simulink model "IEEE9-WT-PV"  (R2024a)
settings: Solver=FixedStepDiscrete  StartTime=0.0  StopTime=Tend  RelTol=1e-3
values from neighbouring files (symbols this model uses):
  beta_0 = 0    [data_WT.m]
  C_4 = 0.1670*C_b    (= 1.00487241952e-06)    [main.m]
  C_6 = 0.2835*C_b    (= 1.70587623314e-06)    [main.m]
  C_8 = 0.2275*C_b    (= 1.36891302659e-06)    [main.m]
  C_dc = 2*S_LV_base*H_DC_base/V_dc_base^2    (= 0.478267523722)    [data_WT.m]    (also in main.m = 1.6)
  C_f = C_f_pu*C_LV_base    (= 0.001461477898)    [data_WT.m]    (also in main.m = 0.00530516476973)
  f_b = 50    [data_WT.m]    (also in main.m)
  fdr_m = 0.05    [main.m]
  fdr_q = 0.01    [main.m]
  G_diff = ss(c2d(s/(20e-3/3*s+1),T_s_cont,'tustin'))    [data_WT.m]
  G_lowpass_disc = ss(c2d(G_lowpass,T_s_cont,'tustin'))    [data_WT.m]
  G_lowpass_disc_1khz = ss(c2d(G_lowpass_1khz,T_s_cont,'tustin'))    [data_WT.m]
  G_setpoint_lowpass_disc = ss(c2d(ss(1/(0.1*s+1)),T_s_cont,'tustin'))    [main.m]
  G_sm_dis = ss(c2d(G_cont_sm,T_s_sim,'tustin'))    [main.m]
  GSC_theta0 = -45.0572/180*pi*0-60/180*pi    (= -1.0471975512)    [data_WT.m]
  I0_total1 = Npar1*I0    (= 7.7895e-08)    [data_PV.m]
  I_GSC_base = S_GSC_base/V_LV_base    (= 30303.030303)    [data_WT.m]
  I_PMSG_0 = T_park(0)^-1*[Z_PMSG^-1*V_LV_base*sqrt(2/3)*([cos(RSC_theta0);sin(RSC_theta0)]-[cos(PMSG_theta0);sin(PMSG_theta0)]);0]    [data_WT.m]
  IL_total1 = Npar1*IL    (= 50459)    [data_PV.m]
  Ipv_scmax1 = Npar1*Ipv_sc    (= 50300)    [data_PV.m]
  island_q = [-0.1312   -0.0230   -0.0343]    [main.m]
  island_Vdc = [1 1.2853    Vpv_mppmax2/Vdc_n]    [main.m]
  island_Vdc_r = [1 1.3430 1.4716]    [main.m]
  island_Vm = [1 1 1]    [main.m]
  J_PMSG_WT_MS = 2*H_PMSGWT_LS*S_PMSG_base/(2*pi*f_b)^2    (= 630.526507942)    [data_WT.m]
  k_p_GSC = 0.02    [data_WT.m]
  k_p_MSC = k_p_GSC    (= 0.02)    [data_WT.m]
  k_theta_GSC = 0.1    [data_WT.m]
  k_theta_MSC = 2/0.6    (= 3.33333333333)    [data_WT.m]
  K_WT_ff_i = 1    [main.m]
  K_WT_ff_v = 1    [main.m]
  K_WT_i_i = 0.79    [main.m]
  K_WT_i_v = 0.69    [main.m]
  K_WT_p_i = 2.1    [main.m]
  K_WT_p_v = 0.15    [main.m]
  Kff_v = 1    [main.m]
  Kffpv_i = 1    [main.m]
  Kp_beta = 270*0    (= 0)    [data_WT.m]
  Kpvi_i1 = Ki_i*Vpv_m/Ipv_b_LV    [main.m]
  Kpvi_v1 = Ki_v*Ipv_b_LV/Vpv_m    [main.m]
  Kpvp_i1 = Kp_i*Vpv_m/Ipv_b_LV    [main.m]
  Kpvp_v1 = Kp_v*Ipv_b_LV/Vpv_m    [main.m]
  L1_pu = 1*0.0186/m    (= 0.000186)    [main.m]
  L_45 = L_lines(2)    [main.m]
  L_56 = L_lines(3)    [main.m]
  L_67 = L_lines(5)    [main.m]
  L_78 = L_lines(6)    [main.m]
  L_89 = L_lines(8)    [main.m]
  L_94 = L_lines(9)    [main.m]
  L_f = L_f_pu*L_LV_base    (= 3.46639466054e-05)    [data_WT.m]    (also in main.m = 9.54929658551e-06)
  L_PMSG = L_PMSG_PU*L_LV_base    (= 3.46639466054e-05)    [data_WT.m]
  main_p = 0.575    [main.m]
  mpv_dc1 = fdr*kg1*w_b/Vdc_n    [main.m]
  mpv_dc1_r = fdr*kg1_r*w_b/Vdc_n    [main.m]
  mpv_p1 = fdr_p/Vdc_n*w_b    [main.m]
  mpv_q1 = fdr_q*Vpv_m/S_b    [main.m]
  Notch_w_10khz = ss(c2d((s^2+w0_f10khz^2)/(s^2+w0_f10khz/Q_f10khz*s+w0_f10khz^2),T_s_sim,'tustin'))    [data_WT.m]
  omega_base = 2*pi*f_b    (= 314.159265359)    [data_WT.m]    (also in main.m)
  omega_wt = 1.4    [data_WT.m]
  R1_pu = 1*0.00734/m    (= 7.34e-05)    [main.m]
  R_45 = R_lines(2)    [main.m]
  R_56 = R_lines(3)    [main.m]
  R_67 = R_lines(5)    [main.m]
  R_78 = R_lines(6)    [main.m]
  R_89 = R_lines(8)    [main.m]
  R_94 = R_lines(9)    [main.m]
  R_f = R_f_pu*Z_LV_base    (= 0.001089)    [data_WT.m]    (also in main.m = 0.0003)
  R_PMSG = R_PMSG_PU*Z_LV_base    (= 0.005445)    [data_WT.m]
  Rpvs_total1 = Rpv_s*Nser1/Npar1    (= 0.0067482)    [data_PV.m]
  RSC_theta0 = 180/180*pi    (= 3.14159265359)    [data_WT.m]
  Rss1 = Vpv_ocmax1/(IL_total1-I0_total1*(exp(Vpv_ocmax1/VT_total1) -1))    [data_PV.m]
  S_b = 100*(10^6)    (= 100000000)    [main.m]
  S_bt = S_b    (= 100000000)    [main.m]
  S_GSC_base = S_LV_base    (= 100000000)    [data_WT.m]
  S_PMSG_base = S_WTPMSG_base    (= 100000000)    [data_WT.m]
  T_load = 20    [main.m]
  T_pitch_servo = 0.5    [data_WT.m]
  T_redispatch = 25    [main.m]
  T_s_cont = 1e-4    (= 0.0001)    [data_WT.m]
  T_s_sim = 1e-7    (= 1e-07)    [data_WT.m]
  V1_rms = 1000    [main.m]
  V2_rms = 13800    [main.m]
  V_dc_base = 7.92e3    (= 7920)    [data_WT.m]
  V_LV_base = 3.3e3    (= 3300)    [data_WT.m]
  V_m = sqrt(2/3)*V1_rms    [main.m]
  v_wind = 12    [data_WT.m]
  Vdc_n = 3*V_m    [main.m]
  Vpv_mppmax1 = Nser1*Vpv_mpp    (= 2945.7)    [data_PV.m]
  Vpv_ocmax1 = Nser1*Vpv_oc    (= 3671.1)    [data_PV.m]
  VT_total1 = VT*Nser1    (= 135.150894483)    [data_PV.m]
  w_b = 2*pi*f_b    (= 314.159265359)    [data_WT.m]    (also in main.m)
undefined symbols (not defined in the file or in its folder): D1, Delta, DiscIntNeverNeededParam, i_dc, PI_pitch
libraries: spsThreePhaseVIMeasurementLib x15, spsThreePhaseSeriesRLCBranchLib x11, spsabctodq0Lib x8, spsThreePhaseTransformerTwoWindingsLib x5, spsThreePhaseParallelRLCLoadLib x5, spsGroundLib x5, spsSeriesRLCBranchLib x5, spsCurrentMeasurementLib x5, spsVoltageMeasurementLib x4, spsPower3phInstantaneousLib x4, spsdq0toabcLib x4, spsThreePhaseParallelRLCBranchLib x3
(part 1 of 3)
settings Model: SimulationMode=accelerator  ExtModeTrigDuration=100  Creator=TayyebiA  LastModifiedBy=dominic
settings SolverCC: AlgebraicLoopSolver=LineSearch
settings DataIOCC: SaveOutput=off  SignalLogging=off  DSMLogging=off  SaveTime=off  ReturnWorkspaceOutputs=off  StateSaveName=tmp_raccel_xout  SignalLoggingName=tmp_raccel_logsout
settings OptimizationCC: EfficientMapNaN2IntZero=off
settings DebuggingCC: UnconnectedInputMsg=warning  UnconnectedOutputMsg=warning  UnconnectedLineMsg=warning  ArithmeticOperatorsInVariantConditions=warning
settings HardwareCC: TargetBitPerLong=64  TargetBitPerPointer=64  TargetBitPerSizeT=64  TargetBitPerPtrDiffT=64  TargetLongLongMode=on  TargetIntDivRoundTo=Zero  TargetEndianess=LittleEndian  TargetWordSize=64  TargetHWDeviceType=MATLAB Host  ProdEqTarget=off
settings ModelReferenceCC: EnableRefExpFcnMdlSchedulingChecks=on
settings SFSimCC: SimUseLocalCustomCode=off  CustomCodeUndefinedFunction=UseInterfaceOnly
settings RTWCC: SystemTargetFile=raccel.tlc  TemplateMakefile=raccel_default_tmf  RTWVerbose=off  RTWUseLocalCustomCode=off  RTWUseSimCustomCode=on  GPUComputeCapability=3.5
settings CodeAppCC: GenerateComments=off  MaxIdLength=128  MangleLength=10  SimulinkBlockComments=off
settings RaccelTargetCC: TargetLangStandard=C99 (ISO)  InstructionSetFMA=off  OptimizeReductions=off  LogToMDFFile=off  ENABLE_SLEXEC_SSBRIDGE=1  RTWCAPIParams=on  RTWCAPIRootIO=off

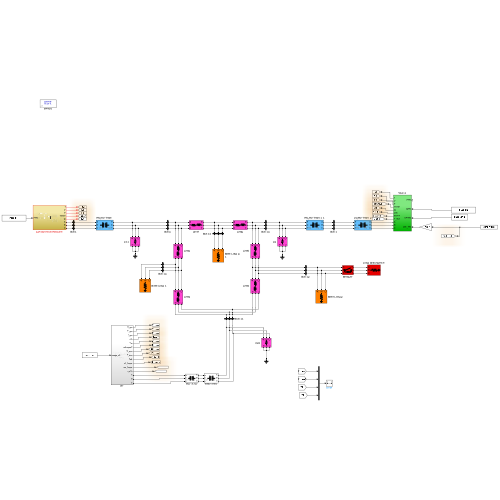
[thumbnail: Simulink's stored preview of the top-level diagram]
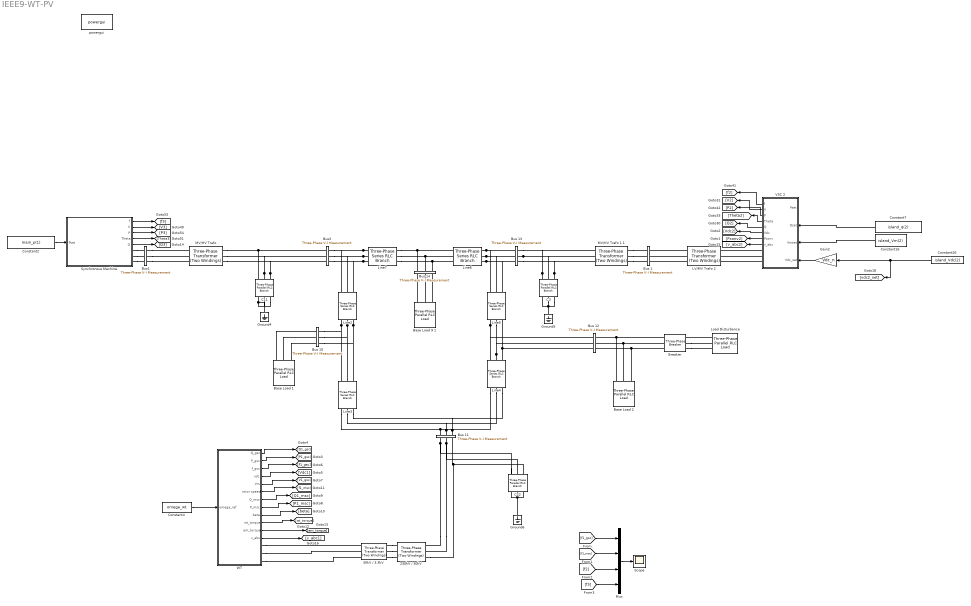
== system IEEE9-WT-PV ==
  230kV / 30kV : spsThreePhaseTransformerTwoWindingsLib/Three-Phase Transformer (Two Windings)  Winding1Connection=Yg  Winding2Connection=Delta (D1)  CoreType=Three single-phase transformers  SetSaturation=off  Hysteresis=off  DataFile='hysteresis'  SetInitialFlux=off  Measurements=None  UNITS=pu  NominalPower=[ 110e6 , f_b ]  Winding1=[ 230e3 , 0.002 , 0.08 ]  Winding2=[ 30e3 , 0.002 , 0.08 ]  Rm=500  Lm=500  L0=0.5  Saturation=[ 0,0 ; 0.0024,1.2 ; 1.0,1.52 ]  InitialFluxes=[ 0.8 , -0.8 , 0.7 ]  BreakLoop=off  DiscreteSolver=Trapezoidal robust  DataType=off  TransfoNumber=1
  30kV / 3.3kV : spsThreePhaseTransformerTwoWindingsLib/Three-Phase Transformer (Two Windings)  Winding1Connection=Yg  Winding2Connection=Delta (D1)  CoreType=Three single-phase transformers  SetSaturation=off  Hysteresis=off  DataFile='hysteresis'  SetInitialFlux=off  Measurements=None  UNITS=pu  NominalPower=[ 110e6 , f_b ]  Winding1=[ 30e3 , 0.002 , 0.08 ]  Winding2=[ 3.3e3 , 0.002 , 0.08 ]  Rm=500  Lm=500  L0=0.5  Saturation=[ 0,0 ; 0.0024,1.2 ; 1.0,1.52 ]  InitialFluxes=[ 0.8 , -0.8 , 0.7 ]  BreakLoop=off  DiscreteSolver=Trapezoidal robust  DataType=off  TransfoNumber=1
  Base Load 1 : spsThreePhaseParallelRLCLoadLib/Three-Phase Parallel RLC Load  LConnTagsString=A|B|C  Configuration=Y (grounded)  NominalVoltage=230e3  Vabc=[1e3 1e3 1e3]  Vabcp=[1e3 1e3 1e3]  NominalFrequency=50  UnbalancedPower=off  ActivePower=pl_island  InductivePower=0  CapacitivePower=0  Pabc=[10e3 9e3 11e3]  QLabc=[100 90 110]  QCabc=[100 90 110]  Pabcp=[10e3 9e3 11e3]  QLabcp=[100 90 110]  QCabcp=[100 90 110]  Measurements=None  LoadType=constant Z
  Base Load 2 : spsThreePhaseParallelRLCLoadLib/Three-Phase Parallel RLC Load  LConnTagsString=A|B|C  Configuration=Y (grounded)  NominalVoltage=230e3  Vabc=[1e3 1e3 1e3]  Vabcp=[1e3 1e3 1e3]  NominalFrequency=50  UnbalancedPower=off  ActivePower=pl_island  InductivePower=0  CapacitivePower=0  Pabc=[10e3 9e3 11e3]  QLabc=[100 90 110]  QCabc=[100 90 110]  Pabcp=[10e3 9e3 11e3]  QLabcp=[100 90 110]  QCabcp=[100 90 110]  Measurements=None  LoadType=constant Z
  Base Load 9 1 : spsThreePhaseParallelRLCLoadLib/Three-Phase Parallel RLC Load  LConnTagsString=A|B|C  Configuration=Y (grounded)  NominalVoltage=230e3  Vabc=[1e3 1e3 1e3]  Vabcp=[1e3 1e3 1e3]  NominalFrequency=50  UnbalancedPower=off  ActivePower=pl_island  InductivePower=0  CapacitivePower=0  Pabc=[10e3 9e3 11e3]  QLabc=[100 90 110]  QCabc=[100 90 110]  Pabcp=[10e3 9e3 11e3]  QLabcp=[100 90 110]  QCabcp=[100 90 110]  Measurements=None  LoadType=constant Z
  Breaker : spsThreePhaseBreakerLib/Three-Phase Breaker  InitialState=open  SwitchA=on  SwitchB=on  SwitchC=on  SwitchTimes=[T_load]  External=off  BreakerResistance=0.01  SnubberResistance=1e6  SnubberCapacitance=inf  Measurements=None
  Bus 1 : spsThreePhaseVIMeasurementLib/Three-Phase V-I Measurement  VoltageMeasurement=no  SetLabelV=on  LabelV=Vabc_8  Vpu=on  VpuLL=off  CurrentMeasurement=no  SetLabelI=on  LabelI=Iabc_8  Ipu=on  Pbase=S_b  Vbase=V_b  OutputType=Complex  PhasorSimulation=off  PSBequivalent=0
  Bus 10 : spsThreePhaseVIMeasurementLib/Three-Phase V-I Measurement  VoltageMeasurement=no  SetLabelV=on  LabelV=Vabc_5  Vpu=on  VpuLL=off  CurrentMeasurement=no  SetLabelI=on  LabelI=Iabc_5  Ipu=on  Pbase=S_b  Vbase=V_b  OutputType=Complex  PhasorSimulation=off  PSBequivalent=0
  Bus 11 : spsThreePhaseVIMeasurementLib/Three-Phase V-I Measurement  VoltageMeasurement=no  SetLabelV=off  LabelV=Vabc_6  Vpu=off  VpuLL=off  CurrentMeasurement=no  SetLabelI=off  LabelI=Iabc_6  Ipu=off  Pbase=S_b  Vbase=V_b  OutputType=Complex  PhasorSimulation=off  PSBequivalent=0
  Bus 12 : spsThreePhaseVIMeasurementLib/Three-Phase V-I Measurement  VoltageMeasurement=no  SetLabelV=on  LabelV=Vabc_5  Vpu=on  VpuLL=off  CurrentMeasurement=no  SetLabelI=on  LabelI=Iabc_5  Ipu=on  Pbase=S_b  Vbase=V_b  OutputType=Complex  PhasorSimulation=off  PSBequivalent=0
  Bus 13 : spsThreePhaseVIMeasurementLib/Three-Phase V-I Measurement  VoltageMeasurement=no  SetLabelV=on  LabelV=Vabc_8  Vpu=on  VpuLL=off  CurrentMeasurement=no  SetLabelI=on  LabelI=Iabc_8  Ipu=on  Pbase=S_b  Vbase=V_b  OutputType=Complex  PhasorSimulation=off  PSBequivalent=0
  Bus 14 : spsThreePhaseVIMeasurementLib/Three-Phase V-I Measurement  VoltageMeasurement=no  SetLabelV=on  LabelV=Vabc_9  Vpu=on  VpuLL=off  CurrentMeasurement=no  SetLabelI=on  LabelI=Iabc_9  Ipu=on  Pbase=S_b  Vbase=V_b  OutputType=Complex  PhasorSimulation=off  PSBequivalent=0
  Bus1 : spsThreePhaseVIMeasurementLib/Three-Phase V-I Measurement  VoltageMeasurement=no  SetLabelV=on  LabelV=Vabc_1  Vpu=on  VpuLL=off  CurrentMeasurement=no  SetLabelI=on  LabelI=Iabc_1  Ipu=on  Pbase=S_b  Vbase=V_b  OutputType=Complex  PhasorSimulation=off  PSBequivalent=0
  Bus3 : spsThreePhaseVIMeasurementLib/Three-Phase V-I Measurement  VoltageMeasurement=no  SetLabelV=on  LabelV=Vabc_4  Vpu=on  VpuLL=off  CurrentMeasurement=no  SetLabelI=on  LabelI=Iabc_4  Ipu=on  Pbase=S_b  Vbase=V_b  OutputType=Complex  PhasorSimulation=off  PSBequivalent=0
  C11 : spsThreePhaseParallelRLCBranchLib/Three-Phase Parallel RLC Branch  LConnTagsString=A|B|C  RConnTagsString=A|B|C  BranchType=C  Resistance=1  Inductance=1e-3  Capacitance=C_4  Measurements=None
  C22 : spsThreePhaseParallelRLCBranchLib/Three-Phase Parallel RLC Branch  LConnTagsString=A|B|C  RConnTagsString=A|B|C  BranchType=C  Resistance=1  Inductance=1e-3  Capacitance=C_6  Measurements=None
  C3 : spsThreePhaseParallelRLCBranchLib/Three-Phase Parallel RLC Branch  LConnTagsString=A|B|C  RConnTagsString=A|B|C  BranchType=C  Resistance=1  Inductance=1e-3  Capacitance=C_8  Measurements=None
  Constant16 : Constant  Value=island_Vm(2)  SampleTime=T_s_cont
  Constant2 : Constant  Value=main_p(1)  SampleTime=T_s_sim
  Constant26 : Constant  Value=island_Vdc(2)  SampleTime=T_s_cont
  Constant4 : Constant  Value=omega_wt  SampleTime=T_s_cont
  Constant7 : Constant  Value=island_q(2)  SampleTime=T_s_cont
  Gain2 : Gain  Gain=Vdc_n
  Ground4 : spsGroundLib/Ground  LConnTagsString=a
  Ground5 : spsGroundLib/Ground  LConnTagsString=a
  Ground6 : spsGroundLib/Ground  LConnTagsString=a
  LV/MV Trafo 2 : spsThreePhaseTransformerTwoWindingsLib/Three-Phase Transformer (Two Windings)  Winding1Connection=Yg  Winding2Connection=Yg  CoreType=Three single-phase transformers  SetSaturation=off  Hysteresis=off  DataFile='hysteresis'  SetInitialFlux=off  Measurements=None  UNITS=pu  NominalPower=[S_bt 50 ]  Winding1="[ V1_rms R1_pu  L1_pu]"  Winding2=[ V2_rms R1_pu L1_pu]  Rm=Rm_pu  Lm=Lm_pu  L0=0.5  Saturation="[ 0,0  ;  0.005,1.2  ;  1.0,1.4 ]"  InitialFluxes=[ 0.8 , -0.8 , 0.7 ]  BreakLoop=off  DiscreteSolver=Trapezoidal robust  DataType=off  TransfoNumber=0
  Line2 : spsThreePhaseSeriesRLCBranchLib/Three-Phase Series RLC Branch  LConnTagsString=A|B|C  RConnTagsString=A|B|C  BranchType=RL  Resistance=R_45  Inductance=L_45  Capacitance=0  Measurements=None
  Line3 : spsThreePhaseSeriesRLCBranchLib/Three-Phase Series RLC Branch  LConnTagsString=A|B|C  RConnTagsString=A|B|C  BranchType=RL  Resistance=R_56  Inductance=L_56  Capacitance=0  Measurements=None
  Line4 : spsThreePhaseSeriesRLCBranchLib/Three-Phase Series RLC Branch  LConnTagsString=A|B|C  RConnTagsString=A|B|C  BranchType=RL  Resistance=R_67  Inductance=L_67  Capacitance=0  Measurements=None
  Line5 : spsThreePhaseSeriesRLCBranchLib/Three-Phase Series RLC Branch  LConnTagsString=A|B|C  RConnTagsString=A|B|C  BranchType=RL  Resistance=R_78  Inductance=L_78  Capacitance=0  Measurements=None
  Line6 : spsThreePhaseSeriesRLCBranchLib/Three-Phase Series RLC Branch  LConnTagsString=A|B|C  RConnTagsString=A|B|C  BranchType=RL  Resistance=R_89  Inductance=L_89  Capacitance=0  Measurements=None
  Line7 : spsThreePhaseSeriesRLCBranchLib/Three-Phase Series RLC Branch  LConnTagsString=A|B|C  RConnTagsString=A|B|C  BranchType=RL  Resistance=R_94  Inductance=L_94  Capacitance=0  Measurements=None
  Load Disturbance : spsThreePhaseParallelRLCLoadLib/Three-Phase Parallel RLC Load  LConnTagsString=A|B|C  Configuration=Y (grounded)  NominalVoltage=230e3  Vabc=[1e3 1e3 1e3]  Vabcp=[1e3 1e3 1e3]  NominalFrequency=50  UnbalancedPower=off  ActivePower=load_step2  InductivePower=0  CapacitivePower=0  Pabc=[10e3 9e3 11e3]  QLabc=[100 90 110]  QCabc=[100 90 110]  Pabcp=[10e3 9e3 11e3]  QLabcp=[100 90 110]  QCabcp=[100 90 110]  Measurements=None  LoadType=constant Z
  "MV/HV Trafo " : spsThreePhaseTransformerTwoWindingsLib/Three-Phase Transformer (Two Windings)  Winding1Connection=Delta (D1)  Winding2Connection=Yg  CoreType=Three single-phase transformers  SetSaturation=off  Hysteresis=off  DataFile='hysteresis'  SetInitialFlux=off  Measurements=None  UNITS=pu  NominalPower=[ 210e6 50 ]  Winding1="[V2_rms 0.0027  0.08]"  Winding2=[230e3 0.0027 0.08]  Rm=500  Lm=500  L0=0.5  Saturation="[ 0,0  ;  0.005,1.2  ;  1.0,1.4 ]"  InitialFluxes=[ 0.8 , -0.8 , 0.7 ]  BreakLoop=off  DiscreteSolver=Trapezoidal robust  DataType=off  TransfoNumber=0
  MV/HV Trafo 1 1 : spsThreePhaseTransformerTwoWindingsLib/Three-Phase Transformer (Two Windings)  Winding1Connection=Yg  Winding2Connection=Yg  CoreType=Three single-phase transformers  SetSaturation=off  Hysteresis=off  DataFile='hysteresis'  SetInitialFlux=off  Measurements=None  UNITS=pu  NominalPower=[ 210e6 50 ]  Winding1=[V2_rms 0.0027 0.08]  Winding2=[230e3 0.0027 0.08]  Rm=500  Lm=500  L0=0.5  Saturation="[ 0,0  ;  0.005,1.2  ;  1.0,1.4 ]"  InitialFluxes=[ 0.8 , -0.8 , 0.7 ]  BreakLoop=off  DiscreteSolver=Trapezoidal robust  DataType=off  TransfoNumber=0
  Mux : Mux
  Scope : Scope
  Synchronous Machine : Subsystem
  VSC 2 : Subsystem
  WT : Subsystem
  powergui : spspowerguiLib/powergui  Priority=1  SimulationMode=Discrete  SampleTime=T_s_sim  frequency=60  Iterations=50  frequencyindice=0  Pbase=100e6  ErrMax=1e-4  UnitsV=kV  UnitsW=MW  buscounter=0  FunctionMessages=off  echomessages=off  EnableUseOfTLC=off  CurrentSourceSwitches=off  DisableSnubberDevices=off  DisableRonSwitches=off  DisableVfSwitches=off  DisplayEquations=off  AutomaticDiscreteSolvers=off  SolverType=Tustin/Backward Euler (TBE)  Interpol=off  ExternalGateDelay=off  methode=off  Ts=100  x0status=blocks  SPID=on  SwTol=0  HookPort=off  NonlinearTolerance=1e-4  nMaxIteration=100  ContinueOnMaxIteration=off  RestoreLinks=warning  ResistiveCurrentMeasurement=off  Frange=[0:2:500]  Ylog=off  Xlog=on  ShowGrid=off  save=off  variable=ZData  structure=0  ZoomFFT=off  StartTime=0.0  cycles=1  DisplayStyle=1  fundamental=60  FreqAxis=off  MaxFrequency=1000  frequencyindicesteady=1  RmsSteady=1  display=off
  wires:
  Synchronous Machine/5(Q) -> [Q3]
  Synchronous Machine/4(Theta) -> [Theta3]
  Synchronous Machine/3(P) -> [P3]
  Synchronous Machine/1(f) -> [f3]
  Synchronous Machine/2(V) -> [V3]
  Constant7/1 -> VSC 2/2(Qset)
  Constant16/1 -> VSC 2/3(Vmset)
  VSC 2/6(Vdc) -> [Vdc2]
  VSC 2/1(f) -> [f2]
  VSC 2/2(V) -> [V2]
  VSC 2/3(P) -> [P2]
  VSC 2/4(Theta) -> [Theta2]
  VSC 2/5(Q) -> [Q2]
  WT/5(Vm) -> [V1_gsc]
  WT/9(beta) -> [beta]
  WT/4(vdc) -> [Vdc1]
  WT/11(em_torque) -> [em_torque]
  WT/10(wt_torque) -> [wt_torque]
  WT/8(P_msc) -> [P1_msc]
  WT/7(Q_msc) -> [Q1_msc]
  WT/6(rotor speed) -> [f1_msc]
  WT/3(f_gsc) -> [f1_gsc]
  WT/2(P_gsc) -> [P1_gsc]
  WT/1(Q_gsc) -> [Q1_gsc]
  Constant2/1 -> Synchronous Machine/1(Pset)
  Constant26/1 -> [vdc2_set], Gain2/1
  Gain2/1 -> VSC 2/4(Vdc_set)
  Constant4/1 -> WT/1(omega_ref)
  VSC 2/7(Pconv) -> [Pconv2]
  VSC 2/8(v_abc) -> [v_abc2]
  WT/12(v_abc) -> [v_abc1]
  [f1_gsc] -> Mux/1
  [f1_msc] -> Mux/2
  [f2] -> Mux/3
  [f3] -> Mux/4
  Mux/1 -> Scope/1
  connections:
  Synchronous Machine/RConn3 -- Bus1/RConn3
  Bus1/LConn3 -- "MV/HV Trafo "/LConn3
  Synchronous Machine/RConn2 -- Bus1/RConn2
  Synchronous Machine/RConn1 -- Bus1/RConn1
  Bus1/LConn2 -- "MV/HV Trafo "/LConn2
  Bus1/LConn1 -- "MV/HV Trafo "/LConn1
  Bus 10/RConn2 -- Base Load 1/LConn2
  Base Load 1/LConn3 -- Bus 10/RConn3
  VSC 2/RConn3 -- LV/MV Trafo 2/LConn3
  VSC 2/RConn2 -- LV/MV Trafo 2/LConn2
  VSC 2/RConn1 -- LV/MV Trafo 2/LConn1
  Bus 12/RConn3 -- Line4/LConn3 -- Line5/RConn3
  Line5/RConn1 -- Bus 12/RConn1 -- Line4/LConn1
  Base Load 1/LConn1 -- Bus 10/RConn1
  Base Load 9 1/LConn2 -- Bus 14/LConn2
  MV/HV Trafo 1 1/LConn3 -- Bus 1/RConn3
  MV/HV Trafo 1 1/LConn1 -- Bus 1/RConn1
  Base Load 9 1/LConn3 -- Bus 14/LConn1
  LV/MV Trafo 2/RConn2 -- Bus 1/LConn2
  LV/MV Trafo 2/RConn3 -- Bus 1/LConn3
  LV/MV Trafo 2/RConn1 -- Bus 1/LConn1
  MV/HV Trafo 1 1/LConn2 -- Bus 1/RConn2
  Base Load 9 1/LConn1 -- Bus 14/LConn3
  C3/LConn3 -- Bus 13/LConn3 -- MV/HV Trafo 1 1/RConn3
  Line7/LConn1 -- Bus3/LConn1 -- Line2/LConn1
  Bus 11/RConn1 -- 230kV / 30kV/LConn1 -- C22/LConn1
  Line6/RConn2 -- Bus 13/RConn2 -- Line5/LConn2
  C22/RConn2 -- C22/RConn3 -- Ground6/LConn1 -- C22/RConn1
  Bus 11/LConn3 -- Line3/RConn3 -- Line4/RConn3
  C11/LConn2 -- Bus3/RConn2 -- "MV/HV Trafo "/RConn2
  Line2/RConn3 -- Line3/LConn3 -- Bus 10/LConn3
  C3/LConn1 -- Bus 13/LConn1 -- MV/HV Trafo 1 1/RConn1
  Line4/LConn2 -- Bus 12/RConn2 -- Line5/RConn2
  Bus 14/RConn2 -- Line7/RConn2 -- Line6/LConn2
  Bus 11/LConn2 -- Line3/RConn2 -- Line4/RConn2
  Line6/RConn1 -- Bus 13/RConn1 -- Line5/LConn1
  C11/LConn1 -- Bus3/RConn1 -- "MV/HV Trafo "/RConn1
  Line7/RConn1 -- Bus 14/RConn3 -- Line6/LConn1
  Line7/RConn3 -- Bus 14/RConn1 -- Line6/LConn3
  C22/LConn3 -- 230kV / 30kV/LConn3 -- Bus 11/RConn3
  Bus 11/RConn2 -- 230kV / 30kV/LConn2 -- C22/LConn2
  Line6/RConn3 -- Bus 13/RConn3 -- Line5/LConn3
  Line7/LConn2 -- Bus3/LConn2 -- Line2/LConn2
  Line2/RConn1 -- Line3/LConn1 -- Bus 10/LConn1
  C3/RConn2 -- C3/RConn3 -- Ground5/LConn1 -- C3/RConn1
  C11/RConn1 -- C11/RConn3 -- Ground4/LConn1 -- C11/RConn2
  Bus 13/LConn2 -- C3/LConn2 -- MV/HV Trafo 1 1/RConn2
  C11/LConn3 -- Bus3/RConn3 -- "MV/HV Trafo "/RConn3
  Line2/RConn2 -- Line3/LConn2 -- Bus 10/LConn2
  Line7/LConn3 -- Bus3/LConn3 -- Line2/LConn3
  Line4/RConn1 -- Line3/RConn1 -- Bus 11/LConn1
  30kV / 3.3kV/LConn2 -- 230kV / 30kV/RConn2
  WT/RConn1 -- 30kV / 3.3kV/RConn1
  30kV / 3.3kV/LConn3 -- 230kV / 30kV/RConn3
  WT/RConn2 -- 30kV / 3.3kV/RConn2
  WT/RConn3 -- 30kV / 3.3kV/RConn3
  30kV / 3.3kV/LConn1 -- 230kV / 30kV/RConn1
  Base Load 2/LConn1 -- Breaker/LConn1 -- Bus 12/LConn1
  Base Load 2/LConn2 -- Bus 12/LConn2 -- Breaker/LConn2
  Base Load 2/LConn3 -- Breaker/LConn3 -- Bus 12/LConn3
  Breaker/RConn3 -- Load Disturbance/LConn3
  Breaker/RConn2 -- Load Disturbance/LConn2
  Load Disturbance/LConn1 -- Breaker/RConn1

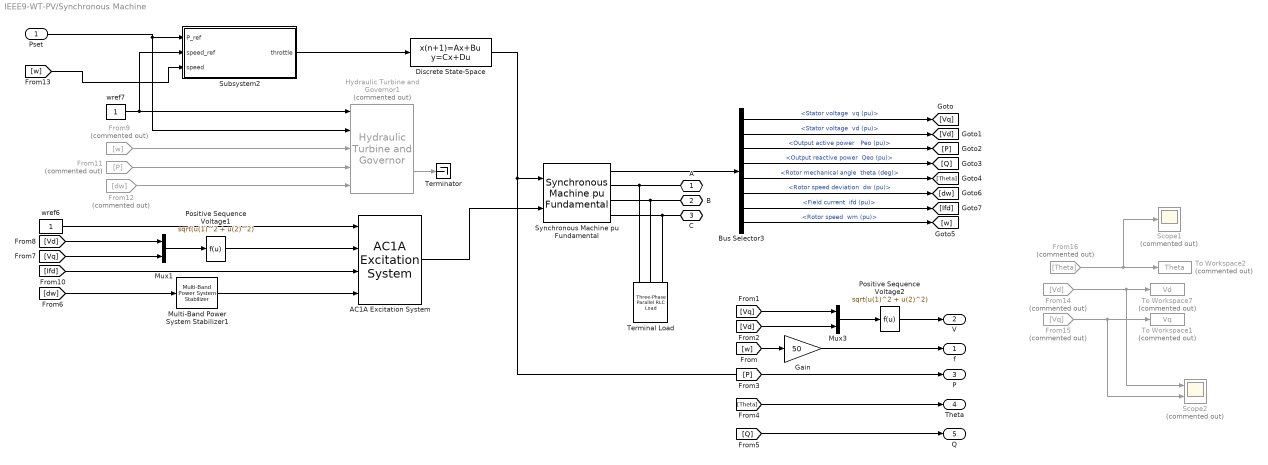
== system IEEE9-WT-PV/Synchronous Machine ==
  Pset : Inport
  AC1A Excitation System : spsAC1AExcitationSystemLib/AC1A Excitation System  Tr=20e-3  KaTa=[400 0.02]  VAminmax=[-14.5 14.5]  VRminmax=[-5.43 6.03]  KfTf=[0.03 1.0]  TbTc=[0 0]  KeTe=[1.0 0.80]  Ve12=[4.18 3.14]  SeVe12=[0.10 0.03]  Kd=0.38  Kc=0.20  v0=[1 1]  TsBlock=T_s_sim
  Bus Selector3 : BusSelector  OutputSignals="dq0 components.Stator voltage  vq (pu),dq0 components.Stator voltage  vd (pu),Output active power   Peo (pu),Output reactive power  Qeo (pu),Mechanical.Rotor mechanical angle  theta (deg),Mechanical.Rotor speed deviation  dw (pu),dq0 components.Field current  ifd (pu),Mechanical.Rotor speed  wm (pu)"
  Discrete State-Space : DiscreteStateSpace  A=G_sm_dis.A  B=G_sm_dis.B  C=G_sm_dis.C  D=G_sm_dis.D  InitialCondition=main_p(1)  SampleTime=T_s_sim
  From11 : From  Commented=on  GotoTag=P
  From12 : From  Commented=on  GotoTag=dw
  From14 : From  Commented=on  GotoTag=Vd
  From15 : From  Commented=on  GotoTag=Vq
  From16 : From  Commented=on  GotoTag=Theta
  From9 : From  Commented=on  GotoTag=w
  Gain : Gain  Gain=50
  Hydraulic Turbine and Governor1 : spsHydraulicTurbineandGovernorLib/Hydraulic Turbine and Governor  Commented=on  sm="[ 10/3  0.07 ]"  gate="[  0.01  0.97518  -0.1  0.1 ]"  reg="[  0.05  1.163  0.105  0  0.01  ]"  hyd="[  0  2.67  ]"  dref=0  po=main_p(1)
  Multi-Band Power System Stabilizer1 : spsMultiBandPowerSystemStabilizerLib/Multi-Band Power System Stabilizer  OperationMode=Simplified settings  Kg=1.0  GL=[0.2 20]  GI=[0.9 25]  GH=[12.0 145]  GLd=[66 66 9.4]  TcLF=[1.667 2 0 0 0 0 2 2.4 0 0 0 0 1 1]  GId=[66 66 47.6]  TcIF=[1 1 0.25 0.3 0 0 1 1 0.3 0.36 0 0 0 0]  GHd=[66 66 233]  TcHF="[0.01 0.012 0 0 0 0  0.012 0.0144 0 0 0 0 1 1]"  LIM=[.075 .15 .15 .15]  Plot_On=off  MagdB_On=off  FreqRange=logspace(-2,2,500)
  Mux1 : Mux  Inputs=2
  Mux3 : Mux  Inputs=2
  Positive Sequence Voltage1 : Fcn  Expr=sqrt(u(1)^2 + u(2)^2)
  Positive Sequence Voltage2 : Fcn  Expr=sqrt(u(1)^2 + u(2)^2)
  Scope1 : Scope  Commented=on
  Scope2 : Scope  Commented=on  NumInputPorts=2
  Subsystem2 : Subsystem
  Synchronous Machine pu Fundamental : spsSynchronousMachinepuFundamentalLib/Synchronous Machine pu Fundamental  PresetModel=No  MechanicalLoad=Mechanical power Pm  ShowDetailedParameters=on  RotorType=Salient-pole  Units=per unit fundamental parameters  MeasurementBus=off  NominalParameters="[100E6  V2_rms   50]"  Stator="[ 2.85E-03  0.114  1.19  0.36 ]"  Field="[ 5.79E-04  0.114]"  Dampers2=[0.0652, 0.5134, 0.0287, 0.2553, 7.765e-3, 0.9167 ]  Dampers1="[ 1.17E-02  0.182  1.97E-02  0.384 ]"  Mechanical=[ 3.7 0 20]  PolePairs=20  InitialConditions="[ 0  0  0  0  0  0  0  0  1 ]"  SetSaturation=off  Saturation=[0.6404,0.7127,0.8441,0.9214,0.9956,1.082,1.19,1.316,1.457;0.7,0.7698,0.8872,0.9466,0.9969,1.046,1.1,1.151,1.201]  LoadFlowParameters=[1,0,0,0,0]  TsPowergui=0  TsBlock=T_s_sim  IterativeModel=Trapezoidal non iterative  IterativeDiscreteModel=Trapezoidal non iterative  BusType=PV  Pref=main_p(1)  Qref=0  Qmin=-inf  Qmax=inf  PLF=0  QLF=0
  Terminal Load : spsThreePhaseParallelRLCLoadLib/Three-Phase Parallel RLC Load  LConnTagsString=A|B|C  Configuration=Y (grounded)  NominalVoltage=V2_rms  Vabc=[1e3 1e3 1e3]  Vabcp=[1e3 1e3 1e3]  NominalFrequency=50  UnbalancedPower=off  ActivePower=500000  InductivePower=0  CapacitivePower=0  Pabc=[10e3 9e3 11e3]  QLabc=[100 90 110]  QCabc=[100 90 110]  Pabcp=[10e3 9e3 11e3]  QLabcp=[100 90 110]  QCabcp=[100 90 110]  Measurements=None  LoadType=constant Z
  Terminator : Terminator
  To Workspace1 : ToWorkspace  Commented=on  VariableName=Vq  SampleTime=T_s_sim
  To Workspace2 : ToWorkspace  Commented=on  VariableName=Theta  SampleTime=T_s_sim
  To Workspace7 : ToWorkspace  Commented=on  VariableName=Vd  SampleTime=T_s_sim
  wref6 : Constant  SampleTime=T_s_sim
  wref7 : Constant  SampleTime=T_s_sim
  A : PMIOPort  Side=Right
  B : PMIOPort  Port=2  Side=Right
  C : PMIOPort  Port=3  Side=Right
  f : Outport  VectorParamsAs1DForOutWhenUnconnected=off
  V : Outport  Port=2  VectorParamsAs1DForOutWhenUnconnected=off
  P : Outport  Port=3  VectorParamsAs1DForOutWhenUnconnected=off
  Theta : Outport  Port=4  VectorParamsAs1DForOutWhenUnconnected=off
  Q : Outport  Port=5  VectorParamsAs1DForOutWhenUnconnected=off
  wires:
  Gain/1 -> f/1
  Positive Sequence Voltage2/1 -> V/1
  Mux3/1 -> Positive Sequence Voltage2/1
  Synchronous Machine pu Fundamental/1 -> Bus Selector3/1
  [w] -> Gain/1
  [Vq] -> Mux3/1
  [Vd] -> Mux3/2
  [Theta] -> Theta/1
  Bus Selector3/1 -> [Vq]  "<Stator voltage  vq (pu)>"
  Bus Selector3/2 -> [Vd]  "<Stator voltage  vd (pu)>"
  Bus Selector3/4 -> [Q]  "<Output reactive power  Qeo (pu)>"
  Bus Selector3/5 -> [Theta]  "<Rotor mechanical angle  theta (deg)>"
  Bus Selector3/6 -> [dw]  "<Rotor speed deviation  dw (pu)>"
  Bus Selector3/7 -> [Ifd]  "<Field current  ifd (pu)>"
  Bus Selector3/8 -> [w]  "<Rotor speed  wm (pu)>"
  [Q] -> Q/1
  From9/1 -> Hydraulic Turbine and Governor1/3
  From11/1 -> Hydraulic Turbine and Governor1/4
  Mux1/1 -> Positive Sequence Voltage1/1
  wref6/1 -> AC1A Excitation System/1
  [Vd] -> Mux1/1
  Hydraulic Turbine and Governor1/2 -> Terminator/1
  wref7/1 -> Hydraulic Turbine and Governor1/1, Subsystem2/2(speed_ref)
  [dw] -> Multi-Band Power System Stabilizer1/1
  From12/1 -> Hydraulic Turbine and Governor1/5
  Pset/1 -> Hydraulic Turbine and Governor1/2, Subsystem2/1(P_ref)
  Multi-Band Power System Stabilizer1/1 -> AC1A Excitation System/4
  AC1A Excitation System/1 -> Synchronous Machine pu Fundamental/2
  [w] -> Subsystem2/3(speed)
  Subsystem2/1(throttle) -> Discrete State-Space/1
  [Vq] -> Mux1/2
  Positive Sequence Voltage1/1 -> AC1A Excitation System/2
  From14/1 -> Scope2/1, To Workspace7/1
  From15/1 -> Scope2/2, To Workspace1/1
  From16/1 -> Scope1/1, To Workspace2/1
  Discrete State-Space/1 -> P/1, Synchronous Machine pu Fundamental/1
  Bus Selector3/3 -> [P]  "<Output active power   Peo (pu)>"
  [Ifd] -> AC1A Excitation System/3
  connections:
  Terminal Load/LConn1 -- Synchronous Machine pu Fundamental/RConn1 -- A/RConn1
  Terminal Load/LConn3 -- Synchronous Machine pu Fundamental/RConn3 -- C/RConn1
  Terminal Load/LConn2 -- Synchronous Machine pu Fundamental/RConn2 -- B/RConn1

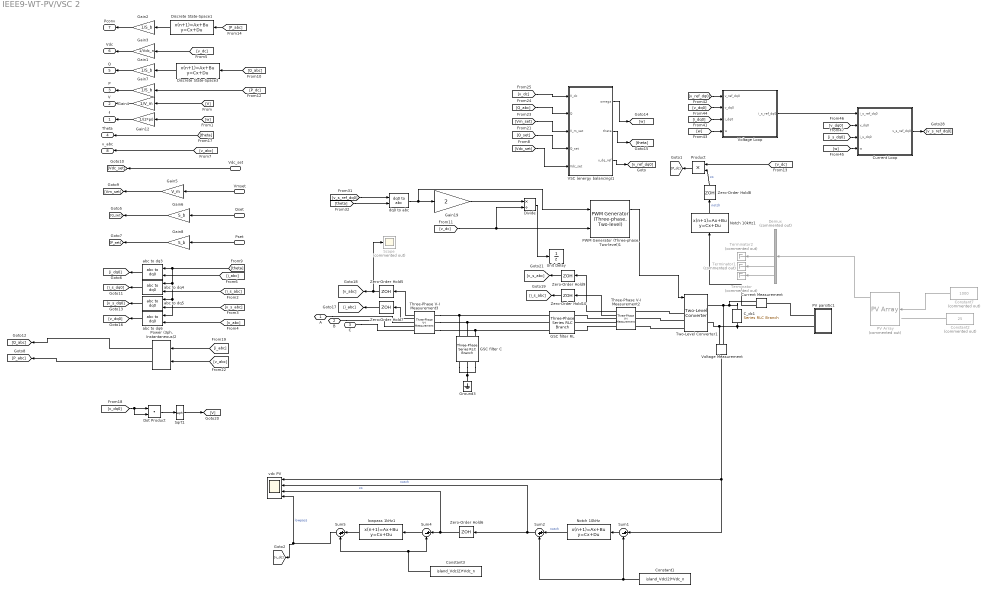
== system IEEE9-WT-PV/VSC 2 ==
  Pset : Inport
  Qset : Inport  Port=2
  Vmset : Inport  Port=3
  Vdc_set : Inport  Port=4
  C_dc1 : spsSeriesRLCBranchLib/Series RLC Branch  LConnTagsString=__new0  RConnTagsString=__new0  BranchType=C  Resistance=1  Inductance=1e-3  SetiL0=off  InitialCurrent=0  Capacitance=C_dc  Setx0=on  InitialVoltage=island_Vdc(2)*Vdc_n  Measurements=None
  Constant1 : Constant  Value=island_Vdc(2)*Vdc_n  SampleTime=T_s_sim
  Constant2 : Constant  Commented=on  Value=25  SampleTime=T_s_sim
  Constant3 : Constant  Value=island_Vdc(2)*Vdc_n  SampleTime=T_s_cont
  Constant7 : Constant  Commented=on  Value=1000  SampleTime=T_s_sim
  Current Loop : Subsystem
  Current Measurement : spsCurrentMeasurementLib/Current Measurement  PhasorSimulation=off  OutputType=Complex  PSBequivalent=0
  Demux : Demux  Commented=on  Outputs=5
  Discrete State-Space1 : DiscreteStateSpace  A=G_lowpass_disc.A  B=G_lowpass_disc.B  C=G_lowpass_disc.C  D=G_lowpass_disc.D  SampleTime=T_s_cont
  Discrete State-Space3 : DiscreteStateSpace  A=G_lowpass_disc.A  B=G_lowpass_disc.B  C=G_lowpass_disc.C  D=G_lowpass_disc.D  SampleTime=T_s_cont
  Divide : Product  Inputs=*/
  Dot Product : DotProduct  OutDataTypeStr=Inherit: Inherit via internal rule
  GSC filter C : spsThreePhaseSeriesRLCBranchLib/Three-Phase Series RLC Branch  LConnTagsString=A|B|C  RConnTagsString=A|B|C  BranchType=C  Resistance=R_f  Inductance=L_f  Capacitance=C_f  Measurements=None
  GSC filter RL : spsThreePhaseSeriesRLCBranchLib/Three-Phase Series RLC Branch  LConnTagsString=A|B|C  RConnTagsString=A|B|C  BranchType=RL  Resistance=R_f  Inductance=L_f  Capacitance=1e-6  Measurements=None
  Gain1 : Gain  Gain=1/S_b
  Gain12 : Gain  Gain=1/(2*pi)
  Gain19 : Gain  Gain=2
  Gain2 : Gain  Gain=1/S_b
  Gain3 : Gain  Gain=1/Vdc_n
  Gain4 : Gain  Gain=1/V_m
  Gain5 : Gain  Gain=V_m
  Gain6 : Gain  Gain=S_b
  Gain7 : Gain  Gain=1/S_b
  Gain8 : Gain  Gain=S_b
  Ground3 : spsGroundLib/Ground  LConnTagsString=a
  Notch 10kHz : DiscreteStateSpace  A=Notch_w_10khz.A  B=Notch_w_10khz.B  C=Notch_w_10khz.C  D=Notch_w_10khz.D  SampleTime=T_s_sim
  Notch 10kHz1 : DiscreteStateSpace  A=Notch_w_10khz.A  B=Notch_w_10khz.B  C=Notch_w_10khz.C  D=Notch_w_10khz.D  SampleTime=T_s_sim
  PV Array : spsPVArrayLib/PV Array  Commented=on  Npar=Npar1  Nser=Nser1  PlotType=array @ 1000 W/m2 & specified temperatures  S_vec="[ 1000  500  100 ]"  Temp_C_vec=[25]  ModuleName=AU Optronics PM060MBR_305W  PlotWhenSelected=off  Pm=305.0436  Ncell=60  Voc=40.79  Isc=10.06  Vm=32.73  Im=9.32  beta_Voc_pc=-0.282  alpha_Isc_pc=0.041998  beta_Voc=-0.11503  alpha_Isc=0.004225  IL=10.0918  I0=1.5579e-11  nI=0.97418  Rsh=118.4621  Rs=0.3749  RobustModel=on  RobustCellTemperature=25  BAL=on  Tc=1e-6  Tfilter=5e-5
  PV parsitic1 : Subsystem
  "PWM Generator (Three-phase, Two-level)1" : eePwmGeneratorTwoLevel/PWM Generator (Three-phase, Two-level)  PWMMode=Continuous PWM (CPWM)  CPWMMode=SPWM: sinusoidal PWM  DPWMMode=60 DPWM: 60 degree discontinuous PWM  fsw=10e3  Ts=T_s_sim
  "Power (3ph, Instantaneous)2" : spsPower3phInstantaneousLib/Power (3ph, Instantaneous)
  Product : Product
  Scope : Scope  Commented=on
  Sqrt1 : Sqrt
  Sum1 : Sum  Inputs=|+-
  Sum2 : Sum  Inputs=|++
  Sum4 : Sum  Inputs=|+-
  Sum5 : Sum  Inputs=|++
  Terminator : Terminator  Commented=on
  Terminator1 : Terminator  Commented=on
  Terminator2 : Terminator  Commented=on
  Three-Phase V-I Measurement2 : spsThreePhaseVIMeasurementLib/Three-Phase V-I Measurement  VoltageMeasurement=phase-to-ground  SetLabelV=off  LabelV=Vabc  Vpu=off  VpuLL=off  CurrentMeasurement=yes  SetLabelI=off  LabelI=Iabc  Ipu=off  Pbase=100e6  Vbase=500e3  OutputType=Complex  PhasorSimulation=off  PSBequivalent=0
  Three-Phase V-I Measurement3 : spsThreePhaseVIMeasurementLib/Three-Phase V-I Measurement  VoltageMeasurement=phase-to-ground  SetLabelV=off  LabelV=Vabc  Vpu=off  VpuLL=off  CurrentMeasurement=yes  SetLabelI=off  LabelI=Iabc  Ipu=off  Pbase=100e6  Vbase=500e3  OutputType=Complex  PhasorSimulation=off  PSBequivalent=0
  Two-Level Converter1 : spsTwoLevelConverterLib/Two-Level Converter  ModelType=Switching devices  Ron=1e-3  Rs=1e6  Cs=inf  Vforward=[0,0]  Ron_Diode=1e-3  Rs_Diode=1e6  Cs_Diode=inf  Vf_Diode=1e-3  Rs_CurrentSource=inf  Ron_ACsource=1e-3
  Unit Delay : UnitDelay  SampleTime=T_s_sim  HasFrameUpgradeWarning=on
  VSC (energy balancing)1 : Subsystem
  Voltage Loop : Subsystem
  Voltage Measurement : spsVoltageMeasurementLib/Voltage Measurement  PhasorSimulation=off  OutputType=Complex  PSBequivalent=0
  Zero-Order Hold{5..10} (6 alike) : ZeroOrderHold  SampleTime=T_s_cont
  abc to dq{3..6} (4 alike) : spsabctodq0Lib/abc to dq0  Alignment=90 degrees behind phase A axis
  dq0 to abc : spsdq0toabcLib/dq0 to abc  Alignment=90 degrees behind phase A axis
  lowpass 1kHz1 : DiscreteStateSpace  A=G_lowpass_disc_1khz.A  B=G_lowpass_disc_1khz.B  C=G_lowpass_disc_1khz.C  D=G_lowpass_disc_1khz.D  SampleTime=T_s_cont
  vdc PV : Scope  NumInputPorts=4
  A : PMIOPort  Side=Right
  B : PMIOPort  Port=2  Side=Right
  C : PMIOPort  Port=3  Side=Right
  f : Outport  VectorParamsAs1DForOutWhenUnconnected=off
  V : Outport  Port=2  VectorParamsAs1DForOutWhenUnconnected=off
  P : Outport  Port=3  VectorParamsAs1DForOutWhenUnconnected=off
  Theta : Outport  Port=4  VectorParamsAs1DForOutWhenUnconnected=off
  Q : Outport  Port=5  VectorParamsAs1DForOutWhenUnconnected=off
  Vdc : Outport  Port=6  VectorParamsAs1DForOutWhenUnconnected=off
  Pconv : Outport  Port=7  VectorParamsAs1DForOutWhenUnconnected=off
  v_abc : Outport  Port=8  VectorParamsAs1DForOutWhenUnconnected=off
  wires:
  Gain7/1 -> P/1
  [V] -> Gain4/1
  Gain12/1 -> f/1
  [w] -> Gain12/1
  Gain4/1 -> V/1
  [theta] -> Theta/1
  [theta] -> abc to dq4/2, abc to dq5/2, abc to dq6/2, abc to dq3/2
  abc to dq3/1 -> [i_dq0]
  abc to dq4/1 -> [i_s_dq0]
  abc to dq5/1 -> [v_s_dq0]
  abc to dq6/1 -> [v_dq0]
  Gain1/1 -> Q/1
  [Q_abc] -> Discrete State-Space3/1
  [v_dc] -> Gain3/1
  Gain3/1 -> Vdc/1
  Vmset/1 -> Gain5/1
  Qset/1 -> Gain6/1
  Pset/1 -> Gain8/1
  Dot Product/1 -> Sqrt1/1
  [v_dq0] -> Dot Product/2, Dot Product/1
  Sqrt1/1 -> [V]
  VSC (energy balancing)1/1(omega) -> [w]
  VSC (energy balancing)1/2(theta) -> [theta]
  [Vdc_set] -> VSC (energy balancing)1/5(Vdc_set)
  [Q_set] -> VSC (energy balancing)1/4(Q_set)
  [Vm_set] -> VSC (energy balancing)1/3(V_m_set)
  [Q_abc] -> VSC (energy balancing)1/2(Q)
  [v_dc] -> VSC (energy balancing)1/1(V_dc)
  Three-Phase V-I Measurement3/1 -> Zero-Order Hold5/1
  Three-Phase V-I Measurement2/1 -> Zero-Order Hold9/1
  Three-Phase V-I Measurement3/2 -> Zero-Order Hold7/1
  Three-Phase V-I Measurement2/2 -> Zero-Order Hold10/1
  Vdc_set/1 -> [Vdc_set]
  Gain5/1 -> [Vm_set]
  Gain6/1 -> [Q_set]
  Gain8/1 -> [P_set]
  [v_ref_dq0] -> Voltage Loop/1(v_ref_dq0)
  [i_s_dq0] -> Current Loop/3(i_s_dq0)
  [v_dq0] -> Current Loop/2(v_dq0)
  Current Loop/1(v_s_ref_dq0) -> [v_s_ref_dq0]
  [w] -> Voltage Loop/4(w)
  [w] -> Current Loop/4(w)
  [theta] -> dq0 to abc/2
  [i_dq0] -> Voltage Loop/3(i_dq0)
  dq0 to abc/1 -> "PWM Generator (Three-phase, Two-level)1"/1, Gain19/1
  [v_s_ref_dq0] -> dq0 to abc/1
  Voltage Loop/1(i_s_ref_dq0) -> Current Loop/1(i_s_ref_dq0)
  [v_dq0] -> Voltage Loop/2(v_dq0)
  Gain19/1 -> Divide/1
  Divide/1 -> Unit Delay/1
  VSC (energy balancing)1/3(v_dq_ref) -> [v_ref_dq0]
  [v_dc] -> Product/1
  Product/1 -> [P_dc]
  [i_abc] -> abc to dq3/1
  [i_s_abc] -> abc to dq4/1
  [v_s_abc] -> abc to dq5/1
  [v_abc] -> abc to dq6/1
  Sum2/1 -> Zero-Order Hold6/1, vdc PV/2  "notch"
  lowpass 1kHz1/1 -> Sum5/1
  Constant1/1 -> Sum2/2, Sum1/2
  Constant3/1 -> Sum4/2, Sum5/2
  Notch 10kHz/1 -> Sum2/1  "notch"
  Sum1/1 -> Notch 10kHz/1
  Sum5/1 -> [v_dc], vdc PV/4  "lowpass"
  Sum4/1 -> lowpass 1kHz1/1
  [v_dc] -> "PWM Generator (Three-phase, Two-level)1"/2, Divide/2
  [i_abc] -> "Power (3ph, Instantaneous)2"/2
  [v_abc] -> "Power (3ph, Instantaneous)2"/1
  Constant7/1 -> PV Array/1
  Notch 10kHz1/1 -> Zero-Order Hold8/1  "notch"
  Zero-Order Hold8/1 -> Product/2  "zo"
  Demux/5 -> Terminator/1
  Demux/4 -> Terminator1/1
  Demux/3 -> Terminator2/1
  PV Array/1 -> Demux/1
  "Power (3ph, Instantaneous)2"/2 -> [Q_abc]
  "Power (3ph, Instantaneous)2"/1 -> [P_abc]
  [P_abc] -> Discrete State-Space1/1
  Gain2/1 -> Pconv/1
  Voltage Measurement/1 -> Sum1/1, vdc PV/1
  Current Measurement/1 -> Notch 10kHz1/1
  Zero-Order Hold6/1 -> vdc PV/3, Sum4/1  "zo"
  Discrete State-Space1/1 -> Gain2/1
  Discrete State-Space3/1 -> Gain1/1
  [P_dc] -> Gain7/1
  Constant2/1 -> ?
  "PWM Generator (Three-phase, Two-level)1"/1 -> Two-Level Converter1/1
  Zero-Order Hold5/1 -> Scope/1, [v_abc]
  Zero-Order Hold7/1 -> [i_abc]
  Zero-Order Hold9/1 -> [v_s_abc]
  Zero-Order Hold10/1 -> [i_s_abc]
  [v_abc] -> v_abc/1
  connections:
  C_dc1/LConn1 -- Current Measurement/RConn1 -- Voltage Measurement/LConn1 -- Two-Level Converter1/RConn1
  C_dc1/RConn1 -- Two-Level Converter1/RConn2 -- Voltage Measurement/LConn2 -- PV parsitic1/RConn2
  Three-Phase V-I Measurement3/LConn2 -- GSC filter C/LConn2 -- GSC filter RL/LConn2
  Three-Phase V-I Measurement3/LConn3 -- GSC filter C/LConn3 -- GSC filter RL/LConn3
  Ground3/LConn1 -- GSC filter C/RConn3 -- GSC filter C/RConn1 -- GSC filter C/RConn2
  Three-Phase V-I Measurement3/LConn1 -- GSC filter C/LConn1 -- GSC filter RL/LConn1
  B/RConn1 -- Three-Phase V-I Measurement3/RConn2
  Three-Phase V-I Measurement2/RConn2 -- GSC filter RL/RConn2
  A/RConn1 -- Three-Phase V-I Measurement3/RConn1
  C/RConn1 -- Three-Phase V-I Measurement3/RConn3
  Three-Phase V-I Measurement2/RConn3 -- GSC filter RL/RConn3
  Three-Phase V-I Measurement2/RConn1 -- GSC filter RL/RConn1
  Two-Level Converter1/LConn1 -- Three-Phase V-I Measurement2/LConn1
  Two-Level Converter1/LConn2 -- Three-Phase V-I Measurement2/LConn2
  Two-Level Converter1/LConn3 -- Three-Phase V-I Measurement2/LConn3
  PV parsitic1/RConn1 -- Current Measurement/LConn1
